simulink model "SVPWM_deadtime系列"  (R2018b)
settings: Solver=FixedStepAuto  StartTime=0.0  StopTime=2  FixedStep=1e-6  RelTol=1e-3
undefined symbols (not defined in the file): j, T_deadtime, Ts, Vdc
libraries: simulink x1
settings Model: Creator=Pis  LastModifiedBy=15210
settings DataIOCC: LimitDataPoints=on  InspectSignalLogs=on
settings OptimizationCC: LifeSpan=inf
settings DebuggingCC: AllowSymbolicDim=off  SFUnexpectedBacktrackingDiag=warning  SFNoUnconditionalDefaultTransitionDiag=warning  SFExecutionAtInitializationDiag=none
settings ModelReferenceCC: PropagateSignalLabelsOutOfModel=off
settings SFSimCC: SimUseLocalCustomCode=off
settings RTWCC: RTWUseLocalCustomCode=off
settings CodeAppCC: StateflowObjectComments=on
settings GRTTargetCC: TargetLangStandard=C89/C90 (ANSI)
settings ConfigComp: CovMetricSettings=dw  CovHtmlReporting=on  CovSaveCumulativeToWorkspaceVar=on  CovSaveSingleToWorkspaceVar=on  CovExternalEMLEnable=off
settings SimscapeCC: SimscapeNormalizeSystem=off

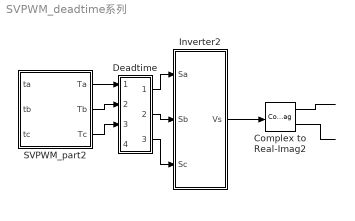
== system SVPWM_deadtime系列 ==
  Complex to Real-Imag2 : ComplexToRealImag
  Deadtime : Subsystem
  Inverter2 : Subsystem
  "SVPWM_part2 " : Subsystem
  wires:
  Complex to Real-Imag2/1 -> ?
  Complex to Real-Imag2/2 -> ?
  Inverter2/1(Vs) -> Complex to Real-Imag2/1
  "SVPWM_part2 "/1(Ta) -> Deadtime/1(ta)
  "SVPWM_part2 "/2(Tb) -> Deadtime/2(tb)
  "SVPWM_part2 "/3(Tc) -> Deadtime/3(tc)
  Deadtime/2(Tb) -> Inverter2/2(Sb)
  Deadtime/1(Ta) -> Inverter2/1(Sa)
  Deadtime/3(Tc) -> Inverter2/3(Sc)

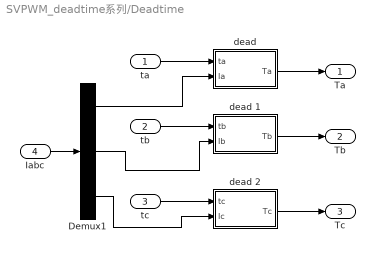
== system SVPWM_deadtime系列/Deadtime ==
  ta : Inport
  tb : Inport  Port=2
  tc : Inport  Port=3
  Iabc : Inport  Port=4
  Demux1 : Demux  Outputs=3
  "dead " : Subsystem
  dead 1 : Subsystem
  dead 2 : Subsystem
  Ta : Outport
  Tb : Outport  Port=2
  Tc : Outport  Port=3
  wires:
  ta/1 -> "dead "/1(ta)
  tb/1 -> dead 1/1(tb)
  tc/1 -> dead 2/1(tc)
  "dead "/1(Ta) -> Ta/1
  dead 1/1(Tb) -> Tb/1
  dead 2/1(Tc) -> Tc/1
  Demux1/1 -> "dead "/2(Ia)
  Demux1/2 -> dead 1/2(Ib)
  Demux1/3 -> dead 2/2(Ic)
  Iabc/1 -> Demux1/1

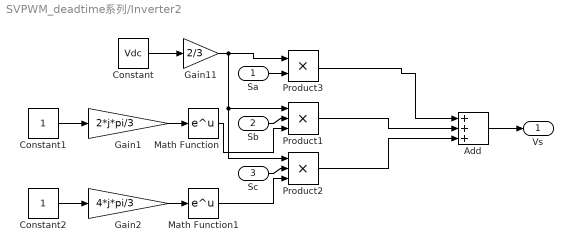
== system SVPWM_deadtime系列/Inverter2 ==
  Sa : Inport
  Sb : Inport  Port=2
  Sc : Inport  Port=3
  Add : Sum  Inputs=+++
  Constant : Constant  Value=Vdc
  Constant1 : Constant
  Constant2 : Constant
  Gain1 : Gain  Gain=2*j*pi/3
  Gain11 : Gain  Gain=2/3
  Gain2 : Gain  Gain=4*j*pi/3
  Math Function : Math  SaturateOnIntegerOverflow=on
  Math Function1 : Math  SaturateOnIntegerOverflow=on
  Product1 : Product  Inputs=3  RndMeth=Zero
  Product2 : Product  Inputs=3  RndMeth=Zero
  Product3 : Product  RndMeth=Zero
  Vs : Outport
  wires:
  Sa/1 -> Product3/2
  Sb/1 -> Product1/2
  Sc/1 -> Product2/2
  Constant/1 -> Gain11/1
  Gain11/1 -> Product2/1, Product1/1, Product3/1
  Product3/1 -> Add/1
  Gain1/1 -> Math Function/1
  Gain2/1 -> Math Function1/1
  Math Function/1 -> Product1/3
  Math Function1/1 -> Product2/3
  Product2/1 -> Add/3
  Constant1/1 -> Gain1/1
  Constant2/1 -> Gain2/1
  Product1/1 -> Add/2
  Add/1 -> Vs/1

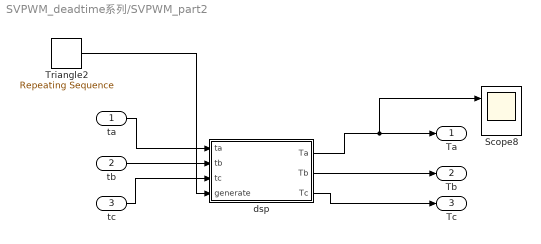
== system SVPWM_deadtime系列/SVPWM_part2  ==
  ta : Inport
  tb : Inport  Port=2
  tc : Inport  Port=3
  Scope8 : Scope  NumInputPorts=2
  Triangle2 : simulink/Sources/Repeating Sequence  rep_seq_t=[0 Ts/2 Ts]  rep_seq_y=[0 1 0]
  dsp : MATLAB Function  TreatAsAtomicUnit=on
  Ta : Outport
  Tb : Outport  Port=2
  Tc : Outport  Port=3
  wires:
  Triangle2/1 -> dsp/4(generate)
  ta/1 -> dsp/1(ta)
  tb/1 -> dsp/2(tb)
  tc/1 -> dsp/3(tc)
  dsp/1(Ta) -> Scope8/1, Ta/1
  dsp/2(Tb) -> Tb/1
  dsp/3(Tc) -> Tc/1

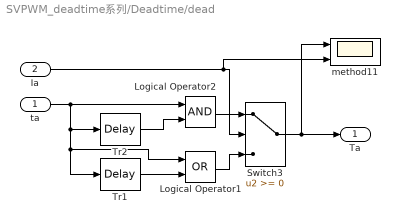
== system SVPWM_deadtime系列/Deadtime/dead  ==
  ta : Inport
  Ia : Inport  Port=2
  Logical Operator1 : Logic  Operator=OR  AllPortsSameDT=off  OutDataTypeStr=boolean
  Logical Operator2 : Logic  AllPortsSameDT=off  OutDataTypeStr=boolean
  Switch3 : Switch
  Tr1 : TransportDelay  DelayTime=T_deadtime
  Tr2 : TransportDelay  DelayTime=T_deadtime
  method11 : Scope  NumInputPorts=2
  Ta : Outport
  wires:
  Tr1/1 -> Logical Operator1/2
  Tr2/1 -> Logical Operator2/2
  Logical Operator2/1 -> Switch3/1
  Logical Operator1/1 -> Switch3/3
  Ia/1 -> method11/2, Switch3/2
  Switch3/1 -> method11/1, Ta/1
  ta/1 -> Tr2/1, Logical Operator1/1, Tr1/1, Logical Operator2/1

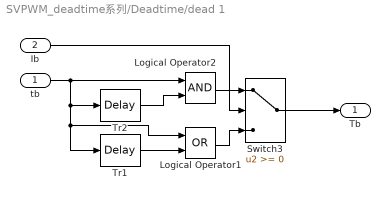
== system SVPWM_deadtime系列/Deadtime/dead 1 ==
  tb : Inport
  Ib : Inport  Port=2
  Logical Operator1 : Logic  Operator=OR  AllPortsSameDT=off  OutDataTypeStr=boolean
  Logical Operator2 : Logic  AllPortsSameDT=off  OutDataTypeStr=boolean
  Switch3 : Switch
  Tr1 : TransportDelay  DelayTime=T_deadtime
  Tr2 : TransportDelay  DelayTime=T_deadtime
  Tb : Outport
  wires:
  Tr1/1 -> Logical Operator1/2
  Tr2/1 -> Logical Operator2/2
  Logical Operator2/1 -> Switch3/1
  Logical Operator1/1 -> Switch3/3
  Ib/1 -> Switch3/2
  Switch3/1 -> Tb/1
  tb/1 -> Tr2/1, Logical Operator1/1, Tr1/1, Logical Operator2/1

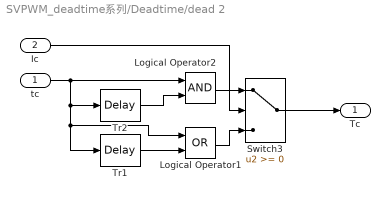
== system SVPWM_deadtime系列/Deadtime/dead 2 ==
  tc : Inport
  Ic : Inport  Port=2
  Logical Operator1 : Logic  Operator=OR  AllPortsSameDT=off  OutDataTypeStr=boolean
  Logical Operator2 : Logic  AllPortsSameDT=off  OutDataTypeStr=boolean
  Switch3 : Switch
  Tr1 : TransportDelay  DelayTime=T_deadtime
  Tr2 : TransportDelay  DelayTime=T_deadtime
  Tc : Outport
  wires:
  Tr1/1 -> Logical Operator1/2
  Tr2/1 -> Logical Operator2/2
  Logical Operator2/1 -> Switch3/1
  Logical Operator1/1 -> Switch3/3
  Ic/1 -> Switch3/2
  Switch3/1 -> Tc/1
  tc/1 -> Tr2/1, Logical Operator1/1, Tr1/1, Logical Operator2/1

== matlab function SVPWM_deadtime系列/SVPWM_part2 /dsp ==
  settings: updateMethod=CONTINUOUS
  data: ta input; Ta output; Tb output; Tc output; tb input; tc input; generate input
function [Ta,Tb,Tc] = fcn(ta,tb,tc,generate)


    X=generate-ta;
    Y=generate-tb;
    Z=generate-tc;
    if (X>=0)
        Ta=1;
    else 
        Ta=0;
    end;
    if (Y>=0)
        Tb=1;
    else 
        Tb=0;
    end;
    if (Z>=0)
        Tc=1;
    else 
        Tc=0;
    end;
